simulink library "MPSV"  (R2025b)
settings: Solver=VariableStepAuto  StartTime=0.0  StopTime=10.0  RelTol=1e-3
undefined symbols (not defined in the file or in its folder): cost, errorCode, goalReached, isFeasible, numberOfPerformedIterations, numPoses, outOfNodes, path, timestampOfComputationUTC
libraries: simulink x31, $bdroot x11, etargetslib x5
(part 2 of 3)

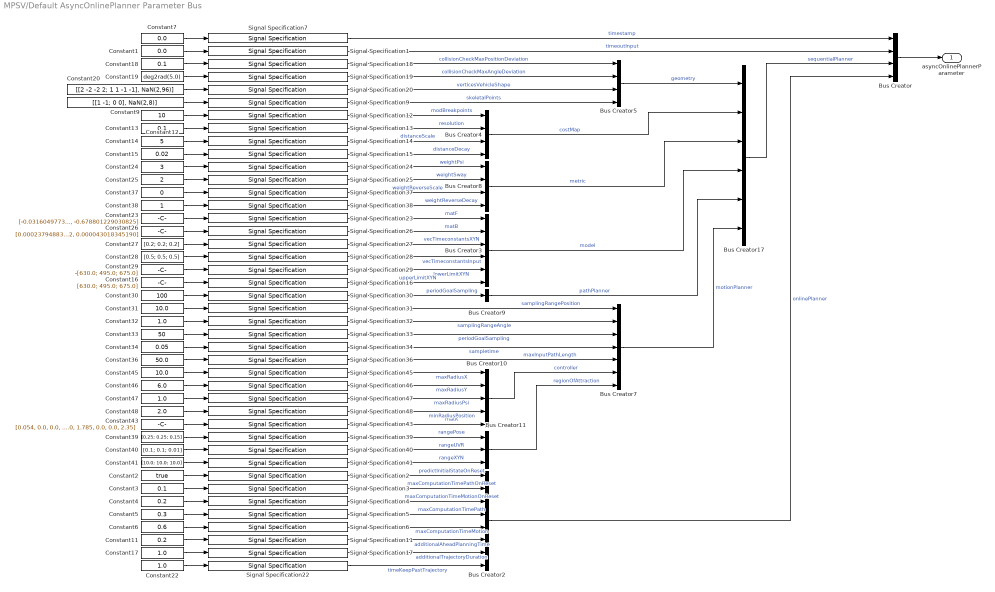
== system MPSV/Default AsyncOnlinePlanner Parameter Bus ==
  Bus Creator{,4..5,8} (4 alike) : BusCreator  Inputs=4
  Bus Creator10 : BusCreator  Inputs=5
  Bus Creator11 : BusCreator  Inputs=3
  Bus Creator17 : BusCreator  Inputs=6
  Bus Creator2 : BusCreator  Inputs=8
  Bus Creator3 : BusCreator  Inputs=6
  Bus Creator7 : BusCreator  Inputs=7
  Bus Creator9 : BusCreator  Inputs=1
  Constant1 : Constant  Value=0.0  OutDataTypeStr=double
  Constant11 : Constant  Value=0.2  OutDataTypeStr=double
  Constant12 : Constant  Value=10  OutDataTypeStr=int32
  Constant13 : Constant  Value=0.1  OutDataTypeStr=double
  Constant14 : Constant  Value=5  OutDataTypeStr=double
  Constant15 : Constant  Value=0.02  OutDataTypeStr=double
  Constant16 : Constant  Value=[630.0; 495.0; 675.0]  OutDataTypeStr=double
  Constant{17,22,32,47} (4 alike) : Constant  Value=1.0  OutDataTypeStr=double
  Constant18 : Constant  Value=0.1  OutDataTypeStr=double
  Constant19 : Constant  Value=deg2rad(5.0)  OutDataTypeStr=double
  Constant2 : Constant  Value=true  OutDataTypeStr=boolean
  Constant20 : Constant  Value=[[2 -2 -2 2; 1 1 -1 -1], NaN(2,96)]  OutDataTypeStr=single
  Constant23 : Constant  Value=[-0.031604977390302, 0.0, 0.0, 0.233741474945168, 0.0, 0.0, 0.0, 0.0, 0.133462292221887, -0.020792892088185, 0.0, 0.0; 0.0, -0.041708610292712, 0.017242263124379, 0.0, -0.251243228165994, -0.000476044356140, 0.0, 0.0, 0.005297185500344, 0.0, -0.167981638498434, 0.497442136687157; 0.0, 0.000017966020615, -0.023528504195578, 0.0, 0.000108223241795, 0.000649602175186, 0.0, 0.0, -0.000002281767319, 0.0, 0.000072358238719, -0.678801229030825]  OutDataTypeStr=double
  Constant24 : Constant  Value=3  OutDataTypeStr=double
  Constant25 : Constant  Value=2  OutDataTypeStr=double
  Constant26 : Constant  Value=[0.000237948834266, -0.000004551592718, 0.000010003488944; -0.000009313932115, 0.000215194147058, -0.000024957572224; -0.000002202124158, -0.000002930260852, 0.000043018345190]  OutDataTypeStr=double
  Constant27 : Constant  Value=[0.2; 0.2; 0.2]  OutDataTypeStr=double
  Constant28 : Constant  Value=[0.5; 0.5; 0.5]  OutDataTypeStr=double
  Constant29 : Constant  Value=-[630.0; 495.0; 675.0]  OutDataTypeStr=double
  Constant3 : Constant  Value=0.1  OutDataTypeStr=double
  Constant30 : Constant  Value=100  OutDataTypeStr=uint32
  Constant31 : Constant  Value=10.0  OutDataTypeStr=double
  Constant33 : Constant  Value=50  OutDataTypeStr=uint32
  Constant34 : Constant  Value=0.05  OutDataTypeStr=double
  Constant36 : Constant  Value=50.0  OutDataTypeStr=double
  Constant37 : Constant  Value=0  OutDataTypeStr=double
  Constant38 : Constant  OutDataTypeStr=double
  Constant39 : Constant  Value=[0.25; 0.25; 0.15]  OutDataTypeStr=double
  Constant4 : Constant  Value=0.2  OutDataTypeStr=double
  Constant40 : Constant  Value=[0.1; 0.1; 0.01]  OutDataTypeStr=double
  Constant41 : Constant  Value=[10.0; 10.0; 10.0]  OutDataTypeStr=double
  Constant43 : Constant  Value=[0.054, 0.0, 0.0, 0.531, 0.0, 0.0, 1.785, 0.0, 0.0, 2.35, 0.0, 0.0; 0.0, 0.054, 0.0, 0.0, 0.531, 0.0, 0.0, 1.785, 0.0, 0.0, 2.35, 0.0; 0.0, 0.0, 0.054, 0.0, 0.0, 0.531, 0.0, 0.0, 1.785, 0.0, 0.0, 2.35]  OutDataTypeStr=double
  Constant45 : Constant  Value=10.0  OutDataTypeStr=double
  Constant46 : Constant  Value=6.0  OutDataTypeStr=double
  Constant48 : Constant  Value=2.0  OutDataTypeStr=double
  Constant5 : Constant  Value=0.3  OutDataTypeStr=double
  Constant6 : Constant  Value=0.6  OutDataTypeStr=double
  Constant7 : Constant  Value=0.0  OutDataTypeStr=double
  Constant9 : Constant  Value=[[1 -1; 0 0], NaN(2,8)]  OutDataTypeStr=single
  Signal Specification{1,3..7,11,17,22,34} (10 alike) : SignalSpecification  OutDataTypeStr=double  Unit=s  Dimensions=1
  Signal Specification12 : SignalSpecification  OutDataTypeStr=int32  Dimensions=1
  Signal Specification{13,18,31,36,45..46,48} (7 alike) : SignalSpecification  OutDataTypeStr=double  Unit=m  Dimensions=1
  Signal Specification{14..15,24..25,37..38} (6 alike) : SignalSpecification  OutDataTypeStr=double  Dimensions=1
  Signal Specification{16,29,39..41} (5 alike) : SignalSpecification  OutDataTypeStr=double  Dimensions=3
  Signal Specification19 : SignalSpecification  OutDataTypeStr=double  Unit=rad  Dimensions=1
  Signal Specification2 : SignalSpecification  OutDataTypeStr=boolean  Dimensions=1
  Signal Specification20 : SignalSpecification  OutDataTypeStr=single  Unit=m  Dimensions=[2,100]
  Signal Specification23 : SignalSpecification  OutDataTypeStr=double  Dimensions=[3,12]
  Signal Specification26 : SignalSpecification  OutDataTypeStr=double  Dimensions=[3,3]
  Signal Specification27 : SignalSpecification  OutDataTypeStr=double  Unit=s  Dimensions=3
  Signal Specification28 : SignalSpecification  OutDataTypeStr=double  Unit=s  Dimensions=3
  Signal Specification30 : SignalSpecification  OutDataTypeStr=uint32  Dimensions=1
  Signal Specification32 : SignalSpecification  OutDataTypeStr=double  Unit=rad  Dimensions=1
  Signal Specification33 : SignalSpecification  OutDataTypeStr=uint32  Dimensions=1
  Signal Specification43 : SignalSpecification  OutDataTypeStr=double  Dimensions=[3,12]
  Signal Specification47 : SignalSpecification  OutDataTypeStr=double  Unit=rad  Dimensions=1
  Signal Specification9 : SignalSpecification  OutDataTypeStr=single  Unit=m  Dimensions=[2,10]
  asyncOnlinePlannerParameter : Outport
  wires:
  Constant24/1 -> Signal Specification24/1
  Constant19/1 -> Signal Specification19/1
  Signal Specification24/1 -> Bus Creator8/1  "weightPsi"
  Bus Creator17/1 -> Bus Creator/3  "sequentialPlanner"
  Constant30/1 -> Signal Specification30/1
  Bus Creator8/1 -> Bus Creator17/3  "metric"
  Constant13/1 -> Signal Specification13/1
  Constant9/1 -> Signal Specification9/1
  Signal Specification25/1 -> Bus Creator8/2  "weightSway"
  Constant18/1 -> Signal Specification18/1
  Constant20/1 -> Signal Specification20/1
  Signal Specification18/1 -> Bus Creator5/1  "collisionCheckMaxPositionDeviation"
  Constant15/1 -> Signal Specification15/1
  Bus Creator4/1 -> Bus Creator17/2  "costMap"
  Signal Specification15/1 -> Bus Creator4/4  "distanceDecay"
  Constant25/1 -> Signal Specification25/1
  Signal Specification19/1 -> Bus Creator5/2  "collisionCheckMaxAngleDeviation"
  Signal Specification12/1 -> Bus Creator4/1  "modBreakpoints"
  Signal Specification20/1 -> Bus Creator5/3  "verticesVehicleShape"
  Bus Creator5/1 -> Bus Creator17/1  "geometry"
  Constant12/1 -> Signal Specification12/1
  Signal Specification14/1 -> Bus Creator4/3  "distanceScale"
  Constant14/1 -> Signal Specification14/1
  Signal Specification13/1 -> Bus Creator4/2  "resolution"
  Bus Creator9/1 -> Bus Creator17/5  "pathPlanner"
  Signal Specification30/1 -> Bus Creator9/1  "periodGoalSampling"
  Signal Specification7/1 -> Bus Creator/1  "timestamp"
  Constant1/1 -> Signal Specification1/1
  Signal Specification1/1 -> Bus Creator/2  "timeoutInput"
  Bus Creator/1 -> asyncOnlinePlannerParameter/1
  Constant2/1 -> Signal Specification2/1
  Signal Specification2/1 -> Bus Creator2/1  "predictInitialStateOnReset"
  Constant3/1 -> Signal Specification3/1
  Constant4/1 -> Signal Specification4/1
  Constant6/1 -> Signal Specification6/1
  Constant5/1 -> Signal Specification5/1
  Constant17/1 -> Signal Specification17/1
  Constant22/1 -> Signal Specification22/1
  Constant11/1 -> Signal Specification11/1
  Signal Specification3/1 -> Bus Creator2/2  "maxComputationTimePathOnReset"
  Signal Specification4/1 -> Bus Creator2/3  "maxComputationTimeMotionOnReset"
  Signal Specification5/1 -> Bus Creator2/4  "maxComputationTimePath"
  Signal Specification6/1 -> Bus Creator2/5  "maxComputationTimeMotion"
  Signal Specification11/1 -> Bus Creator2/6  "additionalAheadPlanningTime"
  Signal Specification17/1 -> Bus Creator2/7  "additionalTrajectoryDuration"
  Signal Specification22/1 -> Bus Creator2/8  "timeKeepPastTrajectory"
  Bus Creator2/1 -> Bus Creator/4  "onlinePlanner"
  Bus Creator3/1 -> Bus Creator17/4  "model"
  Constant23/1 -> Signal Specification23/1
  Signal Specification23/1 -> Bus Creator3/1  "matF"
  Constant26/1 -> Signal Specification26/1
  Signal Specification26/1 -> Bus Creator3/2  "matB"
  Constant27/1 -> Signal Specification27/1
  Signal Specification27/1 -> Bus Creator3/3  "vecTimeconstantsXYN"
  Constant28/1 -> Signal Specification28/1
  Signal Specification28/1 -> Bus Creator3/4  "vecTimeconstantsInput"
  Constant29/1 -> Signal Specification29/1
  Signal Specification29/1 -> Bus Creator3/5  "lowerLimitXYN"
  Bus Creator7/1 -> Bus Creator17/6  "motionPlanner"
  Constant31/1 -> Signal Specification31/1
  Signal Specification31/1 -> Bus Creator7/1  "samplingRangePosition"
  Constant32/1 -> Signal Specification32/1
  Signal Specification32/1 -> Bus Creator7/2  "samplingRangeAngle"
  Constant33/1 -> Signal Specification33/1
  Signal Specification33/1 -> Bus Creator7/3  "periodGoalSampling"
  Constant34/1 -> Signal Specification34/1
  Signal Specification34/1 -> Bus Creator7/4  "sampletime"
  Constant36/1 -> Signal Specification36/1
  Signal Specification36/1 -> Bus Creator7/5  "maxInputPathLength"
  Bus Creator10/1 -> Bus Creator7/6  "controller"
  Bus Creator11/1 -> Bus Creator7/7  "regionOfAttraction"
  Constant39/1 -> Signal Specification39/1
  Signal Specification39/1 -> Bus Creator11/1  "rangePose"
  Constant40/1 -> Signal Specification40/1
  Signal Specification40/1 -> Bus Creator11/2  "rangeUVR"
  Constant41/1 -> Signal Specification41/1
  Signal Specification41/1 -> Bus Creator11/3  "rangeXYN"
  Constant43/1 -> Signal Specification43/1
  Signal Specification43/1 -> Bus Creator10/5  "matK"
  Constant45/1 -> Signal Specification45/1
  Signal Specification45/1 -> Bus Creator10/1  "maxRadiusX"
  Constant46/1 -> Signal Specification46/1
  Signal Specification46/1 -> Bus Creator10/2  "maxRadiusY"
  Constant47/1 -> Signal Specification47/1
  Signal Specification47/1 -> Bus Creator10/3  "maxRadiusPsi"
  Constant48/1 -> Signal Specification48/1
  Signal Specification48/1 -> Bus Creator10/4  "minRadiusPosition"
  Constant7/1 -> Signal Specification7/1
  Constant16/1 -> Signal Specification16/1
  Signal Specification16/1 -> Bus Creator3/6  "upperLimitXYN"
  Constant37/1 -> Signal Specification37/1
  Signal Specification38/1 -> Bus Creator8/4  "weightReverseDecay"
  Signal Specification37/1 -> Bus Creator8/3  "weightReverseScale"
  Constant38/1 -> Signal Specification38/1
  Signal Specification9/1 -> Bus Creator5/4  "skeletalPoints"

== system MPSV/Default PathPlanner Input Bus ==
  Bus Creator : BusCreator  Inputs=6
  Constant1 : Constant  Value=[0;0;0]  OutDataTypeStr=double
  Constant11 : Constant  Value=[0;0;0]  OutDataTypeStr=double
  Constant2 : Constant  Value=[0;0;0]  OutDataTypeStr=double
  Constant22 : Constant  Value=[0;0]  OutDataTypeStr=double
  Constant3 : Constant  Value=[0;0]  OutDataTypeStr=double
  Constant7 : Constant  Value=NaN(2,8000)  OutDataTypeStr=single
  Signal Specification1 : SignalSpecification  OutDataTypeStr=double  Dimensions=3
  Signal Specification11 : SignalSpecification  OutDataTypeStr=double  Dimensions=3
  Signal Specification2 : SignalSpecification  OutDataTypeStr=double  Dimensions=3
  Signal Specification22 : SignalSpecification  OutDataTypeStr=double  Unit=m  Dimensions=2
  Signal Specification3 : SignalSpecification  OutDataTypeStr=double  Unit=m  Dimensions=2
  Signal Specification7 : SignalSpecification  OutDataTypeStr=single  Unit=m  Dimensions=[2,8000]
  pathPlannerInput : Outport
  wires:
  Constant1/1 -> Signal Specification1/1
  Signal Specification1/1 -> Bus Creator/1  "initialPose"
  Constant2/1 -> Signal Specification2/1
  Signal Specification2/1 -> Bus Creator/2  "finalPose"
  Constant3/1 -> Signal Specification3/1
  Signal Specification7/1 -> Bus Creator/6  "verticesStaticObstacles"
  Signal Specification3/1 -> Bus Creator/3  "originOldToNew"
  Bus Creator/1 -> pathPlannerInput/1
  Constant11/1 -> Signal Specification11/1
  Signal Specification11/1 -> Bus Creator/4  "samplingBoxCenterPose"
  Constant22/1 -> Signal Specification22/1
  Signal Specification22/1 -> Bus Creator/5  "samplingBoxDimension"
  Constant7/1 -> Signal Specification7/1

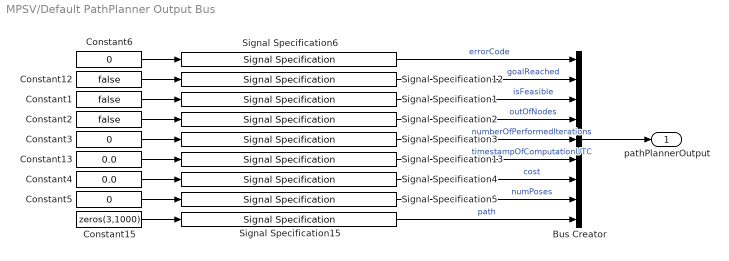
== system MPSV/Default PathPlanner Output Bus ==
  Bus Creator : BusCreator  Inputs=9
  Constant1 : Constant  Value=false  OutDataTypeStr=boolean
  Constant12 : Constant  Value=false  OutDataTypeStr=boolean
  Constant13 : Constant  Value=0.0  OutDataTypeStr=double
  Constant15 : Constant  Value=zeros(3,1000)  OutDataTypeStr=double
  Constant2 : Constant  Value=false  OutDataTypeStr=boolean
  Constant3 : Constant  Value=0  OutDataTypeStr=uint32
  Constant4 : Constant  Value=0.0  OutDataTypeStr=double
  Constant5 : Constant  Value=0  OutDataTypeStr=uint16
  Constant6 : Constant  Value=0  OutDataTypeStr=uint8
  Signal Specification1 : SignalSpecification  OutDataTypeStr=boolean  Dimensions=1
  Signal Specification12 : SignalSpecification  OutDataTypeStr=boolean  Dimensions=1
  Signal Specification13 : SignalSpecification  OutDataTypeStr=double  Unit=s  Dimensions=1
  Signal Specification15 : SignalSpecification  OutDataTypeStr=double  Dimensions=[3,1000]
  Signal Specification2 : SignalSpecification  OutDataTypeStr=boolean  Dimensions=1
  Signal Specification3 : SignalSpecification  OutDataTypeStr=uint32  Dimensions=1
  Signal Specification4 : SignalSpecification  OutDataTypeStr=double  Dimensions=1
  Signal Specification5 : SignalSpecification  OutDataTypeStr=uint16  Dimensions=1
  Signal Specification6 : SignalSpecification  OutDataTypeStr=uint8  Dimensions=1
  pathPlannerOutput : Outport
  wires:
  Signal Specification3/1 -> Bus Creator/5  "numberOfPerformedIterations"
  Signal Specification2/1 -> Bus Creator/4  "outOfNodes"
  Constant1/1 -> Signal Specification1/1
  Constant15/1 -> Signal Specification15/1
  Constant12/1 -> Signal Specification12/1
  Constant13/1 -> Signal Specification13/1
  Constant2/1 -> Signal Specification2/1
  Constant3/1 -> Signal Specification3/1
  Signal Specification1/1 -> Bus Creator/3  "isFeasible"
  Signal Specification12/1 -> Bus Creator/2  "goalReached"
  Signal Specification13/1 -> Bus Creator/6  "timestampOfComputationUTC"
  Signal Specification5/1 -> Bus Creator/8  "numPoses"
  Signal Specification15/1 -> Bus Creator/9  "path"
  Signal Specification4/1 -> Bus Creator/7  "cost"
  Constant5/1 -> Signal Specification5/1
  Constant4/1 -> Signal Specification4/1
  Bus Creator/1 -> pathPlannerOutput/1
  Constant6/1 -> Signal Specification6/1
  Signal Specification6/1 -> Bus Creator/1  "errorCode"

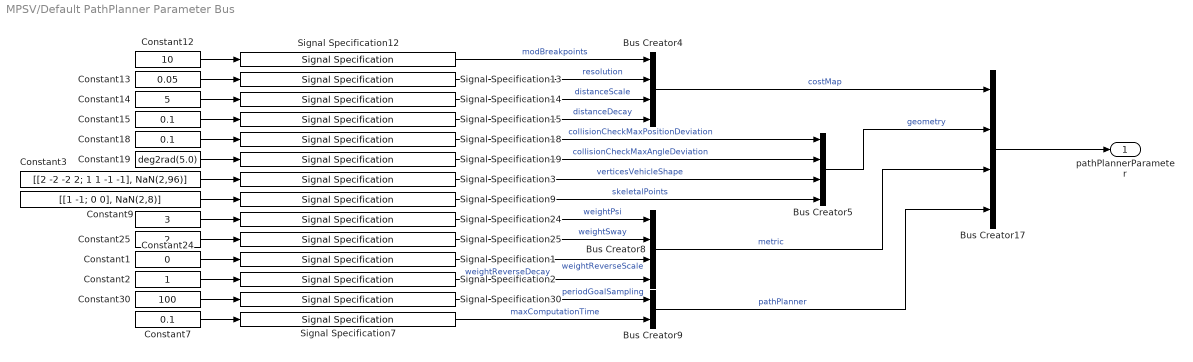
== system MPSV/Default PathPlanner Parameter Bus ==
  Bus Creator{4..5,8,17} (4 alike) : BusCreator  Inputs=4
  Bus Creator9 : BusCreator  Inputs=2
  Constant1 : Constant  Value=0  OutDataTypeStr=double
  Constant12 : Constant  Value=10  OutDataTypeStr=int32
  Constant13 : Constant  Value=0.05  OutDataTypeStr=double
  Constant14 : Constant  Value=5  OutDataTypeStr=double
  Constant15 : Constant  Value=0.1  OutDataTypeStr=double
  Constant18 : Constant  Value=0.1  OutDataTypeStr=double
  Constant19 : Constant  Value=deg2rad(5.0)  OutDataTypeStr=double
  Constant2 : Constant  OutDataTypeStr=double
  Constant24 : Constant  Value=3  OutDataTypeStr=double
  Constant25 : Constant  Value=2  OutDataTypeStr=double
  Constant3 : Constant  Value=[[2 -2 -2 2; 1 1 -1 -1], NaN(2,96)]  OutDataTypeStr=single
  Constant30 : Constant  Value=100  OutDataTypeStr=uint32
  Constant7 : Constant  Value=0.1  OutDataTypeStr=double
  Constant9 : Constant  Value=[[1 -1; 0 0], NaN(2,8)]  OutDataTypeStr=single
  Signal Specification{1..2,14..15,24..25} (6 alike) : SignalSpecification  OutDataTypeStr=double  Dimensions=1
  Signal Specification12 : SignalSpecification  OutDataTypeStr=int32  Dimensions=1
  Signal Specification13 : SignalSpecification  OutDataTypeStr=double  Unit=m  Dimensions=1
  Signal Specification18 : SignalSpecification  OutDataTypeStr=double  Unit=m  Dimensions=1
  Signal Specification19 : SignalSpecification  OutDataTypeStr=double  Unit=rad  Dimensions=1
  Signal Specification3 : SignalSpecification  OutDataTypeStr=single  Unit=m  Dimensions=[2,100]
  Signal Specification30 : SignalSpecification  OutDataTypeStr=uint32  Dimensions=1
  Signal Specification7 : SignalSpecification  OutDataTypeStr=double  Unit=s  Dimensions=1
  Signal Specification9 : SignalSpecification  OutDataTypeStr=single  Unit=m  Dimensions=[2,10]
  pathPlannerParameter : Outport
  wires:
  Signal Specification15/1 -> Bus Creator4/4  "distanceDecay"
  Signal Specification12/1 -> Bus Creator4/1  "modBreakpoints"
  Constant15/1 -> Signal Specification15/1
  Signal Specification13/1 -> Bus Creator4/2  "resolution"
  Bus Creator9/1 -> Bus Creator17/4  "pathPlanner"
  Bus Creator8/1 -> Bus Creator17/3  "metric"
  Constant12/1 -> Signal Specification12/1
  Bus Creator5/1 -> Bus Creator17/2  "geometry"
  Constant18/1 -> Signal Specification18/1
  Constant9/1 -> Signal Specification9/1
  Constant7/1 -> Signal Specification7/1
  Signal Specification14/1 -> Bus Creator4/3  "distanceScale"
  Signal Specification30/1 -> Bus Creator9/1  "periodGoalSampling"
  Constant14/1 -> Signal Specification14/1
  Signal Specification18/1 -> Bus Creator5/1  "collisionCheckMaxPositionDeviation"
  Constant24/1 -> Signal Specification24/1
  Constant13/1 -> Signal Specification13/1
  Signal Specification7/1 -> Bus Creator9/2  "maxComputationTime"
  Constant30/1 -> Signal Specification30/1
  Constant19/1 -> Signal Specification19/1
  Bus Creator4/1 -> Bus Creator17/1  "costMap"
  Signal Specification24/1 -> Bus Creator8/1  "weightPsi"
  Constant25/1 -> Signal Specification25/1
  Signal Specification19/1 -> Bus Creator5/2  "collisionCheckMaxAngleDeviation"
  Signal Specification25/1 -> Bus Creator8/2  "weightSway"
  Bus Creator17/1 -> pathPlannerParameter/1
  Constant1/1 -> Signal Specification1/1
  Constant2/1 -> Signal Specification2/1
  Signal Specification1/1 -> Bus Creator8/3  "weightReverseScale"
  Signal Specification2/1 -> Bus Creator8/4  "weightReverseDecay"
  Constant3/1 -> Signal Specification3/1
  Signal Specification3/1 -> Bus Creator5/3  "verticesVehicleShape"
  Signal Specification9/1 -> Bus Creator5/4  "skeletalPoints"

== system MPSV/Deserialize AsyncOnlinePlanner Output Bus ==
  bytes : Inport  OutDataTypeStr=uint8
  length : Inport  Port=2  OutDataTypeStr=uint32  PortDimensions=1
  AND : Logic  AllPortsSameDT=off  OutDataTypeStr=boolean
  Compare To Constant : simulink/Logic and Bit Operations/Compare To Constant  relop===  const=uint32(52907)  OutDataTypeStr=boolean
  Relational Operator : RelationalOperator  Operator=<=  OutDataTypeStr=boolean  RndMeth=Simplest  InputSameDT=off
  Width : Width  DataType=uint32
  deserialize : Subsystem
  success : Outport  OutDataTypeStr=boolean  PortDimensions=1
  asyncOnlinePlannerOutput : Outport  Port=2
  wires:
  deserialize/1(asyncOnlinePlannerOutput) -> asyncOnlinePlannerOutput/1
  bytes/1 -> Width/1, deserialize/1(bytes)
  length/1 -> Compare To Constant/1, Relational Operator/1
  Compare To Constant/1 -> AND/1
  AND/1 -> deserialize/Enable, success/1
  Relational Operator/1 -> AND/2
  Width/1 -> Relational Operator/2

== system MPSV/PathPlanner ==
  pathPlannerInput : Inport
  pathPlannerParameter : Inport  Port=2
  Deserialize : Subsystem
  SFunctionMPSVPathPlanner : S-Function  FunctionName=SFunctionMPSVPathPlanner  Parameters=SParameter1, SParameter2  SFunctionDeploymentMode=off  EnableBusSupport=off  mask(Legacy Function){SFunctionSpec=void MPSV_PathPlannerStep(void* work1, uint8 y1[24024], uint8 u1[65072]), SParameter1=int16(maxNumNodes), SParameter2=int32(maxNumSamples), ShowSpec=on}
      mask prompts: SParameter1 "P1:"; SParameter2 "P2:"; ShowSpec "Display function specification"
      mask help:
      | This block allows you to call the legacy functions specified by the following Legacy Code Tool definition:
      | def.SFunctionName = 'SFunctionMPSVPathPlanner';
      | def.OutputFcnSpec = 'void MPSV_PathPlannerStep(void* work1, uint8 y1[24024], uint8 u1[65072])';
      | def.StartFcnSpec = 'void MPSV_PathPlannerInitialize(void** work1, int16 p1, uint32 p2)';
      | def.TerminateFcnSpec = 'void MPSV_PathPlannerTerminate(void* work1)';
      | def.HeaderFiles = {'MPSV_DriverPathPlanner.hpp'};
      | def.SourceFiles = {'MPSV_DriverPathPlanner.cpp', 'MPSV_WrapperPathPlanner.cpp'};
      | def.IncPaths = {'code'};
      | def.SrcPaths = {'code'};
      | def.Options.useTlcWithAccel = false;
      mask Help: <p>This block was generated automatically by the Legacy Code Tool. For detailed help on this tool, call<a href="matlab:legacy_code('help')"> legacy_code('help')</a>.</p>
      mask Callback ShowSpec:
      | if strcmp(get_param(gcbh, 'ShowSpec'), 'on')
      |   set_param(gcbh, 'MaskDisplay', sprintf('fprintf(''%s'');', get_param(gcbh, 'SFunctionSpec')));
      | else
      |   set_param(gcbh, 'MaskDisplay', sprintf('fprintf(''%s'');', get_param(gcbh, 'FunctionName')));
      | end
      mask Display: fprintf('void MPSV_PathPlannerStep(void* work1, uint8 y1[24024], uint8 u1[65072])');
  Serialize : Subsystem
  pathPlannerOutput : Outport
  wires:
  pathPlannerInput/1 -> Serialize/1(pathPlannerInput)
  Serialize/1(serializedDataIn) -> SFunctionMPSVPathPlanner/1
  SFunctionMPSVPathPlanner/1 -> Deserialize/1(serializedDataOut)
  Deserialize/1(pathPlannerOutput) -> pathPlannerOutput/1
  pathPlannerParameter/1 -> Serialize/2(pathPlannerParameter)

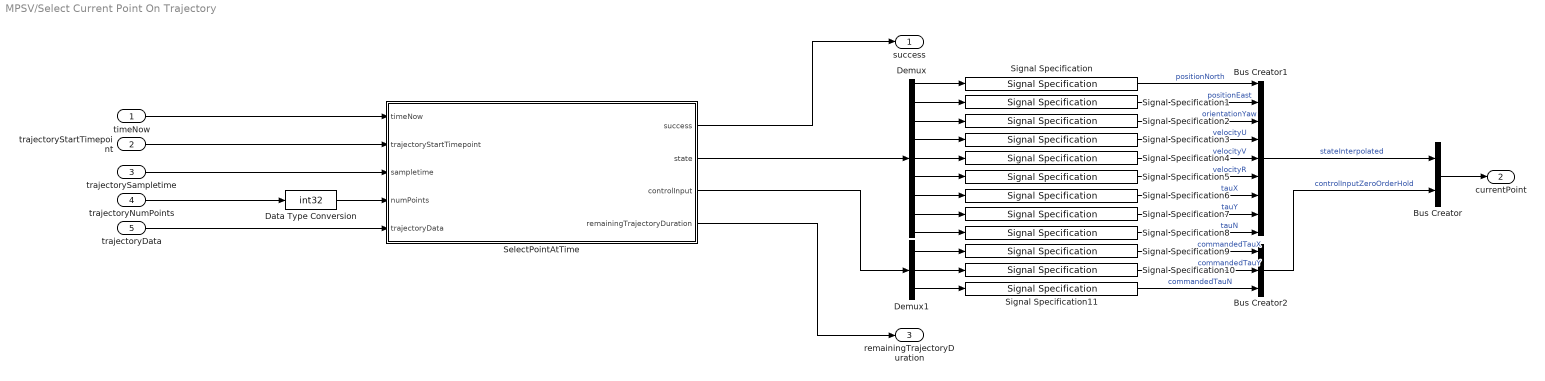
== system MPSV/Select Current Point On Trajectory ==
  timeNow : Inport  OutDataTypeStr=double  Unit=s  PortDimensions=1
  trajectoryStartTimepoint : Inport  Port=2  OutDataTypeStr=double  Unit=s  PortDimensions=1
  trajectorySampletime : Inport  Port=3  OutDataTypeStr=double  Unit=s  PortDimensions=1
  trajectoryNumPoints : Inport  Port=4  PortDimensions=1
  trajectoryData : Inport  Port=5  OutDataTypeStr=double  PortDimensions=[12,500]
  Bus Creator : BusCreator  Inputs=2
  Bus Creator1 : BusCreator  Inputs=9
  Bus Creator2 : BusCreator  Inputs=3
  Data Type Conversion : DataTypeConversion  OutDataTypeStr=int32  SaturateOnIntegerOverflow=off  RndMeth=Floor
  Demux : Demux  Outputs=9
  Demux1 : Demux  Outputs=3
  SelectPointAtTime : MATLAB Function  TreatAsAtomicUnit=on
  Signal Specification : SignalSpecification  OutDataTypeStr=double  Unit=m  Dimensions=1
  Signal Specification1 : SignalSpecification  OutDataTypeStr=double  Unit=m  Dimensions=1
  Signal Specification{6..11} (6 alike) : SignalSpecification  OutDataTypeStr=double  Dimensions=1
  Signal Specification2 : SignalSpecification  OutDataTypeStr=double  Unit=rad  Dimensions=1
  Signal Specification3 : SignalSpecification  OutDataTypeStr=double  Unit=m/s  Dimensions=1
  Signal Specification4 : SignalSpecification  OutDataTypeStr=double  Unit=m/s  Dimensions=1
  Signal Specification5 : SignalSpecification  OutDataTypeStr=double  Unit=rad/s  Dimensions=1
  success : Outport  OutDataTypeStr=boolean  PortDimensions=1
  currentPoint : Outport  Port=2
  remainingTrajectoryDuration : Outport  Port=3  OutDataTypeStr=double  Unit=s  PortDimensions=1
  wires:
  trajectorySampletime/1 -> SelectPointAtTime/3(sampletime)
  trajectoryStartTimepoint/1 -> SelectPointAtTime/2(trajectoryStartTimepoint)
  trajectoryData/1 -> SelectPointAtTime/5(trajectoryData)
  Bus Creator1/1 -> Bus Creator/1  "stateInterpolated"
  Signal Specification5/1 -> Bus Creator1/6  "velocityR"
  Demux/7 -> Signal Specification6/1
  Demux/5 -> Signal Specification4/1
  Signal Specification9/1 -> Bus Creator2/1  "commandedTauX"
  Signal Specification8/1 -> Bus Creator1/9  "tauN"
  Demux/3 -> Signal Specification2/1
  trajectoryNumPoints/1 -> Data Type Conversion/1
  SelectPointAtTime/1(success) -> success/1
  Signal Specification4/1 -> Bus Creator1/5  "velocityV"
  Demux/1 -> Signal Specification/1
  Signal Specification3/1 -> Bus Creator1/4  "velocityU"
  Demux/8 -> Signal Specification7/1
  timeNow/1 -> SelectPointAtTime/1(timeNow)
  Signal Specification7/1 -> Bus Creator1/8  "tauY"
  Data Type Conversion/1 -> SelectPointAtTime/4(numPoints)
  Demux1/3 -> Signal Specification11/1
  Demux1/1 -> Signal Specification9/1
  SelectPointAtTime/2(state) -> Demux/1
  Demux/4 -> Signal Specification3/1
  Signal Specification2/1 -> Bus Creator1/3  "orientationYaw"
  SelectPointAtTime/3(controlInput) -> Demux1/1
  Demux/6 -> Signal Specification5/1
  Signal Specification6/1 -> Bus Creator1/7  "tauX"
  Signal Specification/1 -> Bus Creator1/1  "positionNorth"
  Signal Specification11/1 -> Bus Creator2/3  "commandedTauN"
  Signal Specification10/1 -> Bus Creator2/2  "commandedTauY"
  Signal Specification1/1 -> Bus Creator1/2  "positionEast"
  Demux/9 -> Signal Specification8/1
  Demux1/2 -> Signal Specification10/1
  Demux/2 -> Signal Specification1/1
  Bus Creator2/1 -> Bus Creator/2  "controlInputZeroOrderHold"
  Bus Creator/1 -> currentPoint/1
  SelectPointAtTime/4(remainingTrajectoryDuration) -> remainingTrajectoryDuration/1

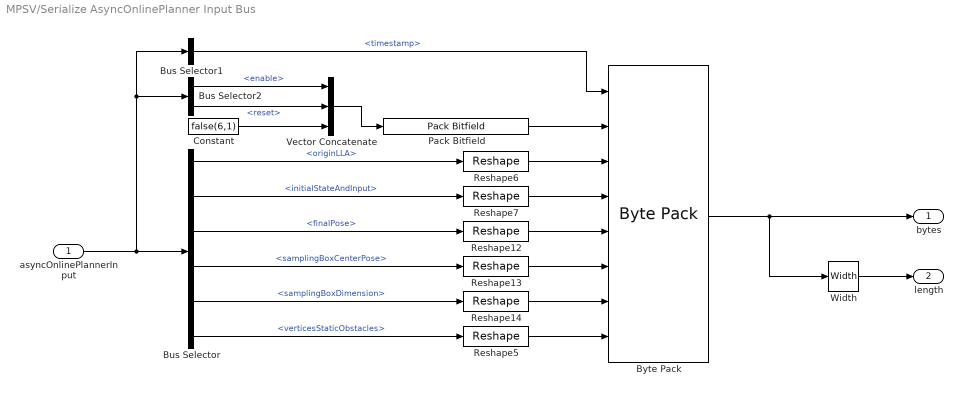
== system MPSV/Serialize AsyncOnlinePlanner Input Bus ==
  asyncOnlinePlannerInput : Inport
  Bus Selector : BusSelector  OutputSignals=originLLA,initialStateAndInput,finalPose,samplingBoxCenterPose,samplingBoxDimension,verticesStaticObstacles
  Bus Selector1 : BusSelector  OutputSignals=timestamp
  Bus Selector2 : BusSelector  OutputSignals=enable,reset
  Byte Pack : etargetslib/Byte Pack  datatypes={'double','uint8','double','double','double','double','double','single'}  byteAlign=1
  Constant : Constant  Value=false(6,1)  OutDataTypeStr=boolean
  Pack Bitfield : $bdroot/details/Pack Bitfield
  Reshape{5..7,12..14} (6 alike) : Reshape
  Vector Concatenate : Concatenate  NumInputs=3
  Width : Width  DataType=uint32
  bytes : Outport  OutDataTypeStr=uint8
  length : Outport  Port=2  OutDataTypeStr=uint32  PortDimensions=1
  wires:
  Byte Pack/1 -> bytes/1, Width/1
  Bus Selector/3 -> Reshape12/1  "<finalPose>"
  Bus Selector/5 -> Reshape14/1  "<samplingBoxDimension>"
  Bus Selector/2 -> Reshape7/1  "<initialStateAndInput>"
  Bus Selector/6 -> Reshape5/1  "<verticesStaticObstacles>"
  Bus Selector/4 -> Reshape13/1  "<samplingBoxCenterPose>"
  Bus Selector/1 -> Reshape6/1  "<originLLA>"
  asyncOnlinePlannerInput/1 -> Bus Selector1/1, Bus Selector2/1, Bus Selector/1
  Width/1 -> length/1
  Bus Selector1/1 -> Byte Pack/1  "<timestamp>"
  Pack Bitfield/1 -> Byte Pack/2
  Reshape14/1 -> Byte Pack/7
  Reshape13/1 -> Byte Pack/6
  Reshape6/1 -> Byte Pack/3
  Reshape7/1 -> Byte Pack/4
  Reshape12/1 -> Byte Pack/5
  Constant/1 -> Vector Concatenate/3
  Vector Concatenate/1 -> Pack Bitfield/1
  Bus Selector2/2 -> Vector Concatenate/2  "<reset>"
  Bus Selector2/1 -> Vector Concatenate/1  "<enable>"
  Reshape5/1 -> Byte Pack/8

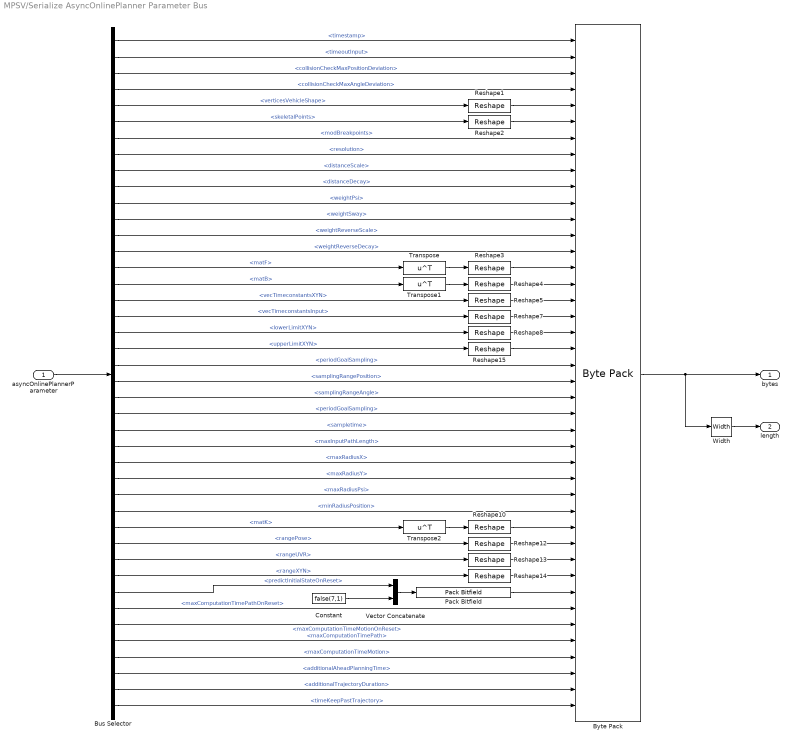
== system MPSV/Serialize AsyncOnlinePlanner Parameter Bus ==
  asyncOnlinePlannerParameter : Inport
  Bus Selector : BusSelector  OutputSignals=timestamp,timeoutInput,sequentialPlanner.geometry.collisionCheckMaxPositionDeviation,sequentialPlanner.geometry.collisionCheckMaxAngleDeviation,sequentialPlanner.geometry.verticesVehicleShape,sequentialPlanner.geometry.skeletalPoints,sequentialPlanner.costMap.modBreakpoints,sequentialPlanner.costMap.resolution,sequentialPlanner.costMap.distanceScale,sequentialPlanner.costMap.distanceDecay,sequentialPlanner.metric.weightPsi,sequentialPlanner.metric.weightSway,sequentialPlanner.metric.weightReverseScale,sequentialPlanner.metric.weightReverseDecay,sequentialPlanner.model.matF,sequentialPlanner.model.matB,sequentialPlanner.model.vecTimeconstantsXYN,sequentialPlanner.model.vecTimeconstantsInput,sequentialPlanner.model.lowerLimitXYN,sequentialPlanner.model.upperLimitXYN,sequentialPlanner.pathPlanner.periodGoalSampling,sequentialPlanner.motionPlanner.samplingRangePosition,sequentialPlanner.motionPlanner.samplingRangeAngle,sequentialPlanner.motionPlanner.periodGoalSampling,sequentialPlanner.motionPlanner.sampletime,sequentialPlanner.motionPlanner.maxInputPathLength,sequentialPlanner.motionPlanner.controller.maxRadiusX,sequentialPlanner.motionPlanner.controller.maxRadiusY,sequentialPlanner.motionPlanner.controller.maxRadiusPsi,sequentialPlanner.motionPlanner.controller.minRadiusPosition,sequentialPlanner.motionPlanner.controller.matK,sequentialPlanner.motionPlanner.regionOfAttraction.rangePose,sequentialPlanner.motionPlanner.regionOfAttraction.rangeUVR,sequentialPlanner.motionPlanner.regionOfAttraction.rangeXYN,onlinePlanner.predictInitialStateOnReset,onlinePlanner.maxComputationTimePathOnReset,onlinePlanner.maxComputationTimeMotionOnReset,onlinePlanner.maxComputationTimePath,onlinePlanner.maxComputationTimeMotion,onlinePlanner.additionalAheadPlanningTime,onlinePlanner.additionalTrajectoryDuration,onlinePlanner.timeKeepPastTrajectory
  Byte Pack : etargetslib/Byte Pack  datatypes={'double','double','double','double','single','single','int32','double','double','double','double','double','double','double','double','double','double','double','double','double','uint32','double','double','uint32','double','double','double','double','double','double','double','double','double','double','uint8','double','double','double','double','double','double','double'}  byteAlign=1
  Constant : Constant  Value=false(7,1)  OutDataTypeStr=boolean
  Pack Bitfield : $bdroot/details/Pack Bitfield
  Reshape{1..5,7..8,10,12..15} (12 alike) : Reshape
  Transpose : Math  Operator=transpose
  Transpose1 : Math  Operator=transpose
  Transpose2 : Math  Operator=transpose
  Vector Concatenate : Concatenate
  Width : Width  DataType=uint32
  bytes : Outport  OutDataTypeStr=uint8
  length : Outport  Port=2  OutDataTypeStr=uint32  PortDimensions=1
  wires:
  Transpose1/1 -> Reshape4/1
  Bus Selector/35 -> Vector Concatenate/1  "<predictInitialStateOnReset>"
  Bus Selector/18 -> Reshape7/1  "<vecTimeconstantsInput>"
  asyncOnlinePlannerParameter/1 -> Bus Selector/1
  Bus Selector/16 -> Transpose1/1  "<matB>"
  Bus Selector/34 -> Reshape14/1  "<rangeXYN>"
  Bus Selector/31 -> Transpose2/1  "<matK>"
  Bus Selector/5 -> Reshape1/1  "<verticesVehicleShape>"
  Bus Selector/33 -> Reshape13/1  "<rangeUVR>"
  Bus Selector/17 -> Reshape5/1  "<vecTimeconstantsXYN>"
  Bus Selector/19 -> Reshape8/1  "<lowerLimitXYN>"
  Transpose2/1 -> Reshape10/1
  Transpose/1 -> Reshape3/1
  Bus Selector/15 -> Transpose/1  "<matF>"
  Bus Selector/32 -> Reshape12/1  "<rangePose>"
  Bus Selector/6 -> Reshape2/1  "<skeletalPoints>"
  Byte Pack/1 -> bytes/1, Width/1
  Width/1 -> length/1
  Constant/1 -> Vector Concatenate/2
  Vector Concatenate/1 -> Pack Bitfield/1
  Bus Selector/20 -> Reshape15/1  "<upperLimitXYN>"
  Bus Selector/1 -> Byte Pack/1  "<timestamp>"
  Bus Selector/2 -> Byte Pack/2  "<timeoutInput>"
  Bus Selector/3 -> Byte Pack/3  "<collisionCheckMaxPositionDeviation>"
  Bus Selector/4 -> Byte Pack/4  "<collisionCheckMaxAngleDeviation>"
  Reshape1/1 -> Byte Pack/5
  Reshape2/1 -> Byte Pack/6
  Bus Selector/7 -> Byte Pack/7  "<modBreakpoints>"
  Bus Selector/8 -> Byte Pack/8  "<resolution>"
  Bus Selector/9 -> Byte Pack/9  "<distanceScale>"
  Bus Selector/10 -> Byte Pack/10  "<distanceDecay>"
  Bus Selector/11 -> Byte Pack/11  "<weightPsi>"
  Bus Selector/12 -> Byte Pack/12  "<weightSway>"
  Bus Selector/13 -> Byte Pack/13  "<weightReverseScale>"
  Bus Selector/14 -> Byte Pack/14  "<weightReverseDecay>"
  Reshape3/1 -> Byte Pack/15
  Reshape4/1 -> Byte Pack/16
  Reshape5/1 -> Byte Pack/17
  Reshape7/1 -> Byte Pack/18
  Reshape8/1 -> Byte Pack/19
  Reshape15/1 -> Byte Pack/20
  Bus Selector/21 -> Byte Pack/21  "<periodGoalSampling>"
  Bus Selector/22 -> Byte Pack/22  "<samplingRangePosition>"
  Bus Selector/23 -> Byte Pack/23  "<samplingRangeAngle>"
  Bus Selector/24 -> Byte Pack/24  "<periodGoalSampling>"
  Bus Selector/25 -> Byte Pack/25  "<sampletime>"
  Bus Selector/26 -> Byte Pack/26  "<maxInputPathLength>"
  Bus Selector/27 -> Byte Pack/27  "<maxRadiusX>"
  Bus Selector/28 -> Byte Pack/28  "<maxRadiusY>"
  Bus Selector/29 -> Byte Pack/29  "<maxRadiusPsi>"
  Bus Selector/30 -> Byte Pack/30  "<minRadiusPosition>"
  Reshape10/1 -> Byte Pack/31
  Reshape12/1 -> Byte Pack/32
  Reshape13/1 -> Byte Pack/33
  Reshape14/1 -> Byte Pack/34
  Pack Bitfield/1 -> Byte Pack/35
  Bus Selector/36 -> Byte Pack/36  "<maxComputationTimePathOnReset>"
  Bus Selector/37 -> Byte Pack/37  "<maxComputationTimeMotionOnReset>"
  Bus Selector/38 -> Byte Pack/38  "<maxComputationTimePath>"
  Bus Selector/39 -> Byte Pack/39  "<maxComputationTimeMotion>"
  Bus Selector/40 -> Byte Pack/40  "<additionalAheadPlanningTime>"
  Bus Selector/41 -> Byte Pack/41  "<additionalTrajectoryDuration>"
  Bus Selector/42 -> Byte Pack/42  "<timeKeepPastTrajectory>"

== system MPSV/details ==
  Pack Bitfield : Subsystem
      mask help: Convert a bitfield of 8 bits to a single byte. The input bitfield must be a vector containing 8 boolean values where the first value indicates whether the LSBit is to be set or not.
      mask DialogControl DescGroupVar Prompt: Pack Bitfield
      mask Display: disp('Pack Bitfield');
  Unpack Bitfield : Subsystem
      mask help: Extract all bits from a single byte. The bitfield output contains 8 boolean values where the first value indicates whether the LSBit is set or not.
      mask DialogControl DescGroupVar Prompt: Unpack Bitfield
      mask Display: disp('Unpack Bitfield');

== system MPSV/AutoTune AsyncOnlinePlanner/Enabled Subsystem ==
  In1 : Inport
  planningParameter : EnablePort
  Out1 : Outport
  wires:
  In1/1 -> Out1/1

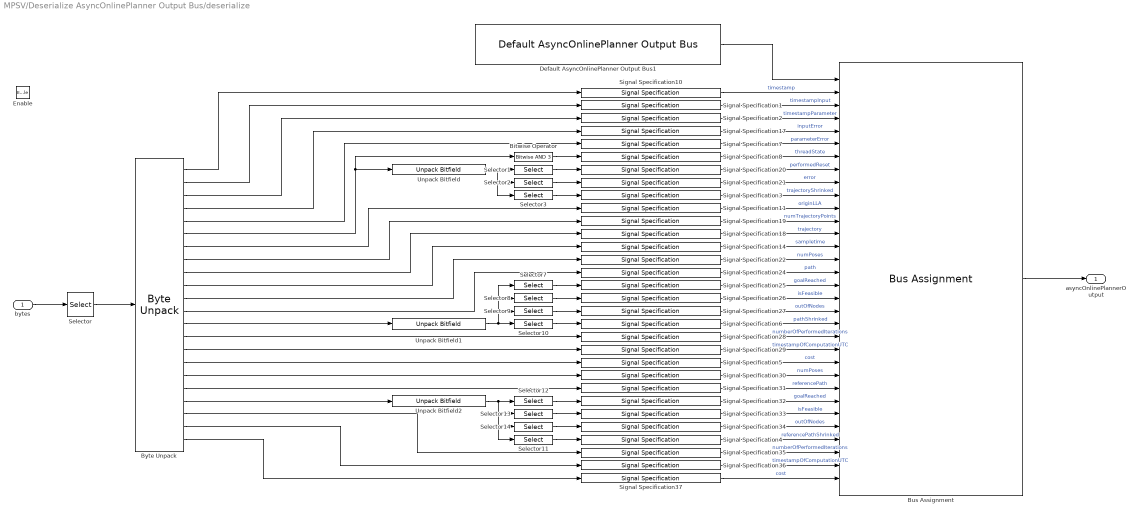
== system MPSV/Deserialize AsyncOnlinePlanner Output Bus/deserialize ==
  bytes : Inport
  Enable : EnablePort
  Bitwise Operator : simulink/Logic and Bit Operations/Bitwise Operator  logicop=AND  UseBitMask=on  BitMask=3  BitMaskRealWorld=Stored Integer
  Bus Assignment : BusAssignment  AssignedSignals=timestamp,timestampInput,timestampParameter,inputError,parameterError,threadState,performedReset,error,trajectoryShrinked,originLLA,numTrajectoryPoints,trajectory,sampletime,pathPlanner.numPoses,pathPlanner.path,pathPlanner.goalReached,pathPlanner.isFeasible,pathPlanner.outOfNodes,pathPlanner.pathShrinked,pathPlanner.numberOfPerformedIterations,pathPlanner.timestampOfComputationUTC,pathPlanner.cost,motionPlanner.numPoses,motionPlanner.referencePath,motionPlanner.goalReached,motionPlanner.isFeasible,motionPlanner.outOfNodes,motionPlanner.referencePathShrinked,motionPlanner.numberOfPerformedIterations,motionPlanner.timestampOfComputationUTC,motionPlanner.cost
  Byte Unpack : etargetslib/Byte Unpack  dimensions={1,1,1,1,1,1,3,1,[12,500],1,1,[3,100],1,1,1,1,1,[3,100],1,1,1,1}  datatypes={'double','double','double','uint8','uint8','uint8','double','uint16','double','double','uint16','double','uint8','uint32','double','double','uint16','double','uint8','uint32','double','double'}  byteAlign=1
      settings: LibrarySourceBlock=embeddedtargetslib/Host Communication/Byte Unpack
  Default AsyncOnlinePlanner Output Bus1 : $bdroot/Default AsyncOnlinePlanner Output Bus
  Selector : Selector  IndexOptions=Index vector (dialog)  Indices=1:52907  OutputSizes=1
  Selector1 : Selector  InputPortWidth=8  IndexOptions=Index vector (dialog)  Indices=3  OutputSizes=1
  Selector10 : Selector  InputPortWidth=8  IndexOptions=Index vector (dialog)  Indices=4  OutputSizes=1
  Selector11 : Selector  InputPortWidth=8  IndexOptions=Index vector (dialog)  Indices=4  OutputSizes=1
  Selector12 : Selector  InputPortWidth=8  IndexOptions=Index vector (dialog)  Indices=1  OutputSizes=1
  Selector13 : Selector  InputPortWidth=8  IndexOptions=Index vector (dialog)  Indices=2  OutputSizes=1
  Selector14 : Selector  InputPortWidth=8  IndexOptions=Index vector (dialog)  Indices=3  OutputSizes=1
  Selector2 : Selector  InputPortWidth=8  IndexOptions=Index vector (dialog)  Indices=4  OutputSizes=1
  Selector3 : Selector  InputPortWidth=8  IndexOptions=Index vector (dialog)  Indices=5  OutputSizes=1
  Selector7 : Selector  InputPortWidth=8  IndexOptions=Index vector (dialog)  Indices=1  OutputSizes=1
  Selector8 : Selector  InputPortWidth=8  IndexOptions=Index vector (dialog)  Indices=2  OutputSizes=1
  Selector9 : Selector  InputPortWidth=8  IndexOptions=Index vector (dialog)  Indices=3  OutputSizes=1
  Signal Specification{1..2,10,14,29,36} (6 alike) : SignalSpecification  OutDataTypeStr=double  Unit=s  Dimensions=1
  Signal Specification11 : SignalSpecification  OutDataTypeStr=double  Dimensions=3
  Signal Specification17 : SignalSpecification  OutDataTypeStr=uint8  Dimensions=1
  Signal Specification18 : SignalSpecification  OutDataTypeStr=double  Dimensions=[12,500]
  Signal Specification19 : SignalSpecification  OutDataTypeStr=uint16  Dimensions=1
  Signal Specification{3..4,6,20..21,25..27,32..34} (11 alike) : SignalSpecification  OutDataTypeStr=boolean  Dimensions=1
  Signal Specification22 : SignalSpecification  OutDataTypeStr=uint16  Dimensions=1
  Signal Specification24 : SignalSpecification  OutDataTypeStr=double  Dimensions=[3,100]
  Signal Specification28 : SignalSpecification  OutDataTypeStr=uint32  Dimensions=1
  Signal Specification30 : SignalSpecification  OutDataTypeStr=uint16  Dimensions=1
  Signal Specification31 : SignalSpecification  OutDataTypeStr=double  Dimensions=[3,100]
  Signal Specification35 : SignalSpecification  OutDataTypeStr=uint32  Dimensions=1
  Signal Specification37 : SignalSpecification  OutDataTypeStr=double  Dimensions=1
  Signal Specification5 : SignalSpecification  OutDataTypeStr=double  Dimensions=1
  Signal Specification7 : SignalSpecification  OutDataTypeStr=uint8  Dimensions=1
  Signal Specification8 : SignalSpecification  OutDataTypeStr=uint8  Dimensions=1
  Unpack Bitfield : $bdroot/details/Unpack Bitfield
  Unpack Bitfield1 : $bdroot/details/Unpack Bitfield
  Unpack Bitfield2 : $bdroot/details/Unpack Bitfield
  asyncOnlinePlannerOutput : Outport
  wires:
  Byte Unpack/2 -> Signal Specification1/1
  Unpack Bitfield2/1 -> Selector14/1, Selector11/1, Selector13/1, Selector12/1
  Signal Specification31/1 -> Bus Assignment/25  "referencePath"
  Byte Unpack/16 -> Signal Specification5/1
  Signal Specification34/1 -> Bus Assignment/28  "outOfNodes"
  Byte Unpack/12 -> Signal Specification24/1
  Selector1/1 -> Signal Specification20/1
  Signal Specification5/1 -> Bus Assignment/23  "cost"
  Byte Unpack/20 -> Signal Specification35/1
  Signal Specification29/1 -> Bus Assignment/22  "timestampOfComputationUTC"
  Unpack Bitfield1/1 -> Selector8/1, Selector7/1, Selector9/1, Selector10/1
  Signal Specification33/1 -> Bus Assignment/27  "isFeasible"
  Bus Assignment/1 -> asyncOnlinePlannerOutput/1
  Unpack Bitfield/1 -> Selector2/1, Selector3/1, Selector1/1
  Bitwise Operator/1 -> Signal Specification8/1
  Selector2/1 -> Signal Specification21/1
  Selector13/1 -> Signal Specification33/1
  Signal Specification25/1 -> Bus Assignment/17  "goalReached"
  Byte Unpack/1 -> Signal Specification10/1
  Byte Unpack/19 -> Unpack Bitfield2/1
  Signal Specification30/1 -> Bus Assignment/24  "numPoses"
  Selector9/1 -> Signal Specification27/1
  Byte Unpack/6 -> Unpack Bitfield/1, Bitwise Operator/1
  Signal Specification37/1 -> Bus Assignment/32  "cost"
  Signal Specification6/1 -> Bus Assignment/20  "pathShrinked"
  Signal Specification28/1 -> Bus Assignment/21  "numberOfPerformedIterations"
  Selector7/1 -> Signal Specification25/1
  Selector/1 -> Byte Unpack/1
  Signal Specification20/1 -> Bus Assignment/8  "performedReset"
  Byte Unpack/21 -> Signal Specification36/1
  Signal Specification36/1 -> Bus Assignment/31  "timestampOfComputationUTC"
  Signal Specification4/1 -> Bus Assignment/29  "referencePathShrinked"
  bytes/1 -> Selector/1
  Signal Specification32/1 -> Bus Assignment/26  "goalReached"
  Signal Specification27/1 -> Bus Assignment/19  "outOfNodes"
  Byte Unpack/22 -> Signal Specification37/1
  Selector14/1 -> Signal Specification34/1
  Signal Specification24/1 -> Bus Assignment/16  "path"
  Signal Specification22/1 -> Bus Assignment/15  "numPoses"
  Byte Unpack/11 -> Signal Specification22/1
  Byte Unpack/17 -> Signal Specification30/1
  Signal Specification26/1 -> Bus Assignment/18  "isFeasible"
  Byte Unpack/13 -> Unpack Bitfield1/1
  Signal Specification35/1 -> Bus Assignment/30  "numberOfPerformedIterations"
  Default AsyncOnlinePlanner Output Bus1/1 -> Bus Assignment/1
  Signal Specification14/1 -> Bus Assignment/14  "sampletime"
  Selector8/1 -> Signal Specification26/1
  Selector11/1 -> Signal Specification4/1
  Byte Unpack/3 -> Signal Specification2/1
  Selector12/1 -> Signal Specification32/1
  Byte Unpack/14 -> Signal Specification28/1
  Selector10/1 -> Signal Specification6/1
  Byte Unpack/18 -> Signal Specification31/1
  Byte Unpack/15 -> Signal Specification29/1
  Byte Unpack/9 -> Signal Specification18/1
  Byte Unpack/7 -> Signal Specification11/1
  Byte Unpack/8 -> Signal Specification19/1
  Byte Unpack/10 -> Signal Specification14/1
  Signal Specification18/1 -> Bus Assignment/13  "trajectory"
  Signal Specification3/1 -> Bus Assignment/10  "trajectoryShrinked"
  Signal Specification11/1 -> Bus Assignment/11  "originLLA"
  Signal Specification10/1 -> Bus Assignment/2  "timestamp"
  Signal Specification19/1 -> Bus Assignment/12  "numTrajectoryPoints"
  Signal Specification8/1 -> Bus Assignment/7  "threadState"
  Signal Specification21/1 -> Bus Assignment/9  "error"
  Signal Specification1/1 -> Bus Assignment/3  "timestampInput"
  Signal Specification2/1 -> Bus Assignment/4  "timestampParameter"
  Selector3/1 -> Signal Specification3/1
  Signal Specification17/1 -> Bus Assignment/5  "inputError"
  Signal Specification7/1 -> Bus Assignment/6  "parameterError"
  Byte Unpack/4 -> Signal Specification17/1
  Byte Unpack/5 -> Signal Specification7/1

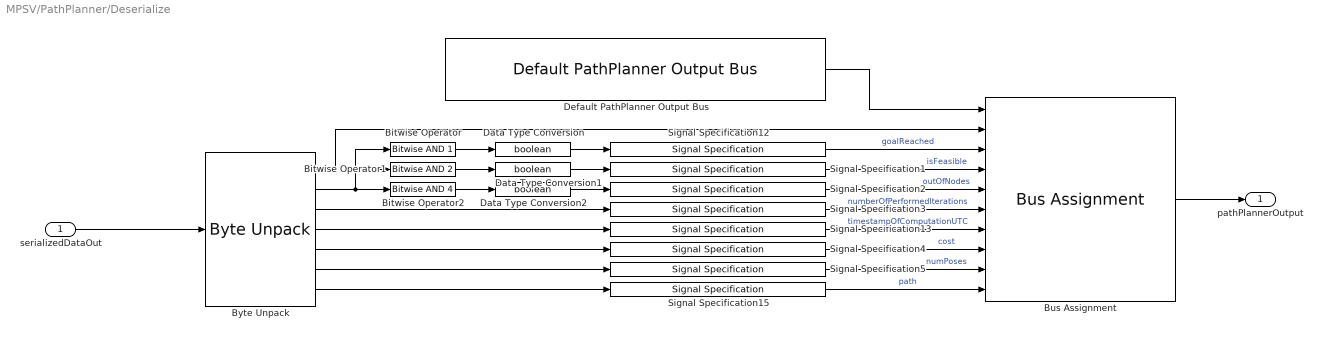
== system MPSV/PathPlanner/Deserialize ==
  serializedDataOut : Inport
  Bitwise Operator : simulink/Logic and Bit Operations/Bitwise Operator  logicop=AND  UseBitMask=on  BitMask=1  BitMaskRealWorld=Stored Integer
  Bitwise Operator1 : simulink/Logic and Bit Operations/Bitwise Operator  logicop=AND  UseBitMask=on  BitMask=2  BitMaskRealWorld=Stored Integer
  Bitwise Operator2 : simulink/Logic and Bit Operations/Bitwise Operator  logicop=AND  UseBitMask=on  BitMask=4  BitMaskRealWorld=Stored Integer
  Bus Assignment : BusAssignment  AssignedSignals=errorCode,goalReached,isFeasible,outOfNodes,numberOfPerformedIterations,timestampOfComputationUTC,cost,numPoses,path
  Byte Unpack : etargetslib/Byte Unpack  dimensions={1,1,1,1,1,1,[3,1000]}  datatypes={'uint8','uint8','uint32','double','double','uint16','double'}  byteAlign=1
      settings: LibrarySourceBlock=embeddedtargetslib/Host Communication/Byte Unpack
  Data Type Conversion : DataTypeConversion  OutDataTypeStr=boolean  SaturateOnIntegerOverflow=off  RndMeth=Floor
  Data Type Conversion1 : DataTypeConversion  OutDataTypeStr=boolean  SaturateOnIntegerOverflow=off  RndMeth=Floor
  Data Type Conversion2 : DataTypeConversion  OutDataTypeStr=boolean  SaturateOnIntegerOverflow=off  RndMeth=Floor
  Default PathPlanner Output Bus : $bdroot/Default PathPlanner Output Bus
  Signal Specification1 : SignalSpecification  OutDataTypeStr=boolean  Dimensions=1
  Signal Specification12 : SignalSpecification  OutDataTypeStr=boolean  Dimensions=1
  Signal Specification13 : SignalSpecification  OutDataTypeStr=double  Unit=s  Dimensions=1
  Signal Specification15 : SignalSpecification  OutDataTypeStr=double  Dimensions=[3,1000]
  Signal Specification2 : SignalSpecification  OutDataTypeStr=boolean  Dimensions=1
  Signal Specification3 : SignalSpecification  OutDataTypeStr=uint32  Dimensions=1
  Signal Specification4 : SignalSpecification  OutDataTypeStr=double  Dimensions=1
  Signal Specification5 : SignalSpecification  OutDataTypeStr=uint16  Dimensions=1
  pathPlannerOutput : Outport
  wires:
  Bitwise Operator1/1 -> Data Type Conversion1/1
  Byte Unpack/2 -> Bitwise Operator/1, Bitwise Operator1/1, Bitwise Operator2/1
  Bitwise Operator2/1 -> Data Type Conversion2/1
  Signal Specification4/1 -> Bus Assignment/8  "cost"
  Signal Specification1/1 -> Bus Assignment/4  "isFeasible"
  Signal Specification2/1 -> Bus Assignment/5  "outOfNodes"
  Byte Unpack/5 -> Signal Specification4/1
  Byte Unpack/3 -> Signal Specification3/1
  Signal Specification3/1 -> Bus Assignment/6  "numberOfPerformedIterations"
  Data Type Conversion/1 -> Signal Specification12/1
  Signal Specification13/1 -> Bus Assignment/7  "timestampOfComputationUTC"
  Byte Unpack/6 -> Signal Specification5/1
  Signal Specification5/1 -> Bus Assignment/9  "numPoses"
  Bitwise Operator/1 -> Data Type Conversion/1
  Signal Specification15/1 -> Bus Assignment/10  "path"
  Data Type Conversion1/1 -> Signal Specification1/1
  Data Type Conversion2/1 -> Signal Specification2/1
  Byte Unpack/4 -> Signal Specification13/1
  Signal Specification12/1 -> Bus Assignment/3  "goalReached"
  Byte Unpack/7 -> Signal Specification15/1
  Default PathPlanner Output Bus/1 -> Bus Assignment/1
  Bus Assignment/1 -> pathPlannerOutput/1
  serializedDataOut/1 -> Byte Unpack/1
  Byte Unpack/1 -> Bus Assignment/2

== system MPSV/PathPlanner/Serialize ==
  pathPlannerInput : Inport
  pathPlannerParameter : Inport  Port=2
  Bus Selector : BusSelector  OutputSignals=initialPose,finalPose,originOldToNew,samplingBoxCenterPose,samplingBoxDimension,verticesStaticObstacles
  Bus Selector1 : BusSelector  OutputSignals=costMap.modBreakpoints,costMap.resolution,costMap.distanceScale,costMap.distanceDecay,geometry.collisionCheckMaxPositionDeviation,geometry.collisionCheckMaxAngleDeviation,geometry.verticesVehicleShape,geometry.skeletalPoints,metric.weightPsi,metric.weightSway,metric.weightReverseScale,metric.weightReverseDecay,pathPlanner.periodGoalSampling,pathPlanner.maxComputationTime
  Byte Pack : etargetslib/Byte Pack  datatypes={'int32','double','double','double','double','double','single','single','double','double','double','double','uint32','double','double','double','double','double','double','single'}  byteAlign=1
  Reshape{1..3,5..9} (8 alike) : Reshape
  serializedDataIn : Outport
  wires:
  Bus Selector/1 -> Reshape1/1  "<initialPose>"
  Bus Selector/6 -> Reshape5/1  "<verticesStaticObstacles>"
  Bus Selector/2 -> Reshape2/1  "<finalPose>"
  Bus Selector/3 -> Reshape3/1  "<originOldToNew>"
  pathPlannerInput/1 -> Bus Selector/1
  Byte Pack/1 -> serializedDataIn/1
  Bus Selector/4 -> Reshape8/1  "<samplingBoxCenterPose>"
  Bus Selector/5 -> Reshape9/1  "<samplingBoxDimension>"
  pathPlannerParameter/1 -> Bus Selector1/1
  Bus Selector1/8 -> Reshape7/1  "<skeletalPoints>"
  Bus Selector1/1 -> Byte Pack/1  "<modBreakpoints>"
  Bus Selector1/2 -> Byte Pack/2  "<resolution>"
  Bus Selector1/3 -> Byte Pack/3  "<distanceScale>"
  Bus Selector1/4 -> Byte Pack/4  "<distanceDecay>"
  Bus Selector1/5 -> Byte Pack/5  "<collisionCheckMaxPositionDeviation>"
  Bus Selector1/6 -> Byte Pack/6  "<collisionCheckMaxAngleDeviation>"
  Bus Selector1/7 -> Reshape6/1  "<verticesVehicleShape>"
  Reshape6/1 -> Byte Pack/7
  Bus Selector1/9 -> Byte Pack/9  "<weightPsi>"
  Bus Selector1/10 -> Byte Pack/10  "<weightSway>"
  Bus Selector1/11 -> Byte Pack/11  "<weightReverseScale>"
  Bus Selector1/12 -> Byte Pack/12  "<weightReverseDecay>"
  Bus Selector1/13 -> Byte Pack/13  "<periodGoalSampling>"
  Bus Selector1/14 -> Byte Pack/14  "<maxComputationTime>"
  Reshape1/1 -> Byte Pack/15
  Reshape2/1 -> Byte Pack/16
  Reshape3/1 -> Byte Pack/17
  Reshape5/1 -> Byte Pack/20
  Reshape8/1 -> Byte Pack/18
  Reshape9/1 -> Byte Pack/19
  Reshape7/1 -> Byte Pack/8

== system MPSV/details/Pack Bitfield ==
  bitfield : Inport  OutDataTypeStr=boolean  PortDimensions=8
  Bitwise Operator : simulink/Logic and Bit Operations/Bitwise Operator  logicop=OR  UseBitMask=off  NumInputPorts=8  BitMask=bin2dec('11011001')  BitMaskRealWorld=Stored Integer
  Data Type Conversion : DataTypeConversion  OutDataTypeStr=uint8  SaturateOnIntegerOverflow=off  RndMeth=Floor
  Demux : Demux  Outputs=8
  Shift Arithmetic : ArithShift  BitShiftNumber=1  BitShiftDirection=Left
  Shift Arithmetic1 : ArithShift  BitShiftNumber=2  BitShiftDirection=Left
  Shift Arithmetic2 : ArithShift  BitShiftNumber=3  BitShiftDirection=Left
  Shift Arithmetic3 : ArithShift  BitShiftNumber=4  BitShiftDirection=Left
  Shift Arithmetic4 : ArithShift  BitShiftNumber=5  BitShiftDirection=Left
  Shift Arithmetic5 : ArithShift  BitShiftNumber=6  BitShiftDirection=Left
  Shift Arithmetic6 : ArithShift  BitShiftNumber=7  BitShiftDirection=Left
  byte : Outport  OutDataTypeStr=uint8  PortDimensions=1
  wires:
  Shift Arithmetic4/1 -> Bitwise Operator/6
  Shift Arithmetic/1 -> Bitwise Operator/2
  Demux/2 -> Shift Arithmetic/1
  Data Type Conversion/1 -> Demux/1
  bitfield/1 -> Data Type Conversion/1
  Demux/6 -> Shift Arithmetic4/1
  Shift Arithmetic5/1 -> Bitwise Operator/7
  Demux/8 -> Shift Arithmetic6/1
  Shift Arithmetic1/1 -> Bitwise Operator/3
  Shift Arithmetic6/1 -> Bitwise Operator/8
  Shift Arithmetic3/1 -> Bitwise Operator/5
  Shift Arithmetic2/1 -> Bitwise Operator/4
  Demux/7 -> Shift Arithmetic5/1
  Demux/3 -> Shift Arithmetic1/1
  Demux/5 -> Shift Arithmetic3/1
  Demux/1 -> Bitwise Operator/1
  Demux/4 -> Shift Arithmetic2/1
  Bitwise Operator/1 -> byte/1
